simulink model "oneaFMModulator"  (R2018a)
settings: Solver=VariableStepAuto  StartTime=0.0  StopTime=0.2  RelTol=1e-3
undefined symbols (not defined in the file): DiscIntNeverNeededParam
libraries: dspsrcs4 x1
settings Model: Creator=Neo  LastModifiedBy=Neo

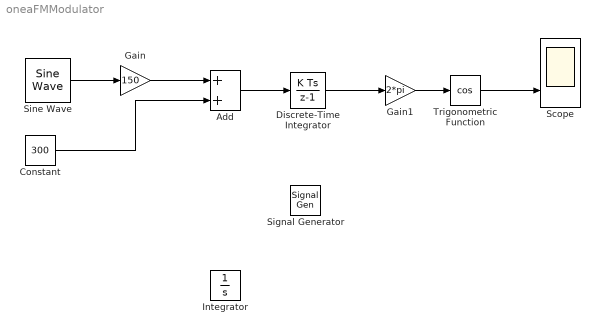
== system oneaFMModulator ==
  Add : Sum
  Constant : Constant  Value=300
  Discrete-Time Integrator : DiscreteIntegrator  SampleTime=1/98000  ICPrevOutput=DiscIntNeverNeededParam  ICPrevScaledInput=DiscIntNeverNeededParam
  Gain : Gain  Gain=150
  Gain1 : Gain  Gain=2*pi
  Integrator : Integrator
  Scope : Scope  NumInputPorts=2
  Signal Generator : SignalGenerator  WaveForm=square  Frequency=10
  Sine Wave : dspsrcs4/Sine Wave  Amplitude=1  Frequency=10  Phase=pi/2  SampleMode=Discrete  OutComplex=Real  CompMethod=Trigonometric fcn  TableSize=Speed  SampleTime=1/98000  SamplesPerFrame=1  ResetState=Restart at time zero  OutputFrames=off  dataType=double  wordLen=16  udDataType=sfix(16)  fracBitsMode=Best precision  numFracBits=15  OutDataTypeStr=double  LastOutDataTypeStr=double
  Trigonometric Function : Trigonometry  Operator=cos
  wires:
  Gain/1 -> Add/1
  Constant/1 -> Add/2
  Gain1/1 -> Trigonometric Function/1
  Trigonometric Function/1 -> Scope/2
  Discrete-Time Integrator/1 -> Gain1/1
  Add/1 -> Discrete-Time Integrator/1
  Sine Wave/1 -> Gain/1
